simulink model "IEEE9Buses"  (R2024b)
settings: Solver=FixedStepAuto  StartTime=0  StopTime=5  FixedStep=1e-6  RelTol=1e-3
values from neighbouring files (symbols this model uses):
  SG_D_1_D = 0.01056    [SG9_parameters.m]
  SG_D_1_EnableSaturation = 0    [SG9_parameters.m]
  SG_D_1_f0 = 60    [SG9_parameters.m]
  SG_D_1_H = 7.5    [SG9_parameters.m]
  SG_D_1_K_A = 20    [SG9_parameters.m]
  SG_D_1_K_E = 1.000000e+1    (= 10)    [SG9_parameters.m]
  SG_D_1_K_F = 2.363    [SG9_parameters.m]
  SG_D_1_K_s = 5    [SG9_parameters.m]
  SG_D_1_R_a = 0.001088    [SG9_parameters.m]
  SG_D_1_S_A = 1    [SG9_parameters.m]
  SG_D_1_S_B = 0.103    [SG9_parameters.m]
  SG_D_1_S_N = 10.659857    [SG9_parameters.m]
  SG_D_1_SpeedPara = 200    [SG9_parameters.m]
  SG_D_1_T_0 = 0.720173    [SG9_parameters.m]
  SG_D_1_T_1 = 0.3    [SG9_parameters.m]
  SG_D_1_T_2 = 0.05    [SG9_parameters.m]
  SG_D_1_T_3 = 0.02    [SG9_parameters.m]
  SG_D_1_T_4 = 0.005    [SG9_parameters.m]
  SG_D_1_T_A = 0.02    [SG9_parameters.m]
  SG_D_1_T_dd = 8.000000e+0    (= 8)    [SG9_parameters.m]
  SG_D_1_T_ddd = 0.04    [SG9_parameters.m]
  SG_D_1_T_E = 0.314    [SG9_parameters.m]
  SG_D_1_T_F = 0.35    [SG9_parameters.m]
  SG_D_1_T_qd = 0.8    [SG9_parameters.m]
  SG_D_1_T_qdd = 0.02    [SG9_parameters.m]
  SG_D_1_T_speed = 0.1    [SG9_parameters.m]
  SG_D_1_T_w = 0.5    [SG9_parameters.m]
  SG_D_1_V_ref = 1.990276    [SG9_parameters.m]
  SG_D_1_w_ref = 376.991118    [SG9_parameters.m]
  SG_D_1_x_d = 1.9    [SG9_parameters.m]
  SG_D_1_x_dd = 0.302    [SG9_parameters.m]
  SG_D_1_x_ddd = 0.204    [SG9_parameters.m]
  SG_D_1_x_l = 0.05    [SG9_parameters.m]
  SG_D_1_x_q = 1.3    [SG9_parameters.m]
  SG_D_1_x_qd = 0.5    [SG9_parameters.m]
  SG_D_1_x_qdd = 0.3    [SG9_parameters.m]
  SG_D_2_D = 0.01056    [SG9_parameters.m]
  SG_D_2_EnableSaturation = 0    [SG9_parameters.m]
  SG_D_2_f0 = 60    [SG9_parameters.m]
  SG_D_2_H = 7.5    [SG9_parameters.m]
  SG_D_2_K_A = 20    [SG9_parameters.m]
  SG_D_2_K_E = 1.000000e+1    (= 10)    [SG9_parameters.m]
  SG_D_2_K_F = 2.363    [SG9_parameters.m]
  SG_D_2_K_s = 0.5    [SG9_parameters.m]
  SG_D_2_R_a = 0.001088    [SG9_parameters.m]
  SG_D_2_S_A = 1    [SG9_parameters.m]
  SG_D_2_S_B = 0.103    [SG9_parameters.m]
  SG_D_2_S_N = 10.659857    [SG9_parameters.m]
  SG_D_2_SpeedPara = 200    [SG9_parameters.m]
  SG_D_2_T_0 = 1.632913    [SG9_parameters.m]
  SG_D_2_T_1 = 0.2    [SG9_parameters.m]
  SG_D_2_T_2 = 0.05    [SG9_parameters.m]
  SG_D_2_T_3 = 0.02    [SG9_parameters.m]
  SG_D_2_T_4 = 0.005    [SG9_parameters.m]
  SG_D_2_T_A = 0.02    [SG9_parameters.m]
  SG_D_2_T_dd = 8.000000e+0    (= 8)    [SG9_parameters.m]
  SG_D_2_T_ddd = 0.04    [SG9_parameters.m]
  SG_D_2_T_E = 0.314    [SG9_parameters.m]
  SG_D_2_T_F = 0.35    [SG9_parameters.m]
  SG_D_2_T_qd = 0.8    [SG9_parameters.m]
  SG_D_2_T_qdd = 0.02    [SG9_parameters.m]
  SG_D_2_T_speed = 0.1    [SG9_parameters.m]
  SG_D_2_T_w = 0.5    [SG9_parameters.m]
  SG_D_2_V_ref = 2.662631    [SG9_parameters.m]
  SG_D_2_w_ref = 376.991118    [SG9_parameters.m]
  SG_D_2_x_d = 1.9    [SG9_parameters.m]
  SG_D_2_x_dd = 0.302    [SG9_parameters.m]
  SG_D_2_x_ddd = 0.204    [SG9_parameters.m]
  SG_D_2_x_l = 0.05    [SG9_parameters.m]
  SG_D_2_x_q = 1.3    [SG9_parameters.m]
  SG_D_2_x_qd = 0.5    [SG9_parameters.m]
  SG_D_2_x_qdd = 0.3    [SG9_parameters.m]
  SG_D_3_D = 0.01056    [SG9_parameters.m]
  SG_D_3_EnableSaturation = 0    [SG9_parameters.m]
  SG_D_3_f0 = 60    [SG9_parameters.m]
  SG_D_3_H = 7.5    [SG9_parameters.m]
  SG_D_3_K_A = 20    [SG9_parameters.m]
  SG_D_3_K_E = 1.000000e+1    (= 10)    [SG9_parameters.m]
  SG_D_3_K_F = 2.363    [SG9_parameters.m]
  SG_D_3_K_s = 0.5    [SG9_parameters.m]
  SG_D_3_R_a = 0.001088    [SG9_parameters.m]
  SG_D_3_S_A = 1    [SG9_parameters.m]
  SG_D_3_S_B = 0.103    [SG9_parameters.m]
  SG_D_3_S_N = 10.659857    [SG9_parameters.m]
  SG_D_3_SpeedPara = 200    [SG9_parameters.m]
  SG_D_3_T_0 = 0.850788    [SG9_parameters.m]
  SG_D_3_T_1 = 0.2    [SG9_parameters.m]
  SG_D_3_T_2 = 0.05    [SG9_parameters.m]
  SG_D_3_T_3 = 0.02    [SG9_parameters.m]
  SG_D_3_T_4 = 0.005    [SG9_parameters.m]
  SG_D_3_T_A = 0.02    [SG9_parameters.m]
  SG_D_3_T_dd = 8.000000e+0    (= 8)    [SG9_parameters.m]
  SG_D_3_T_ddd = 0.04    [SG9_parameters.m]
  SG_D_3_T_E = 0.314    [SG9_parameters.m]
  SG_D_3_T_F = 0.35    [SG9_parameters.m]
  SG_D_3_T_qd = 0.8    [SG9_parameters.m]
  SG_D_3_T_qdd = 0.02    [SG9_parameters.m]
  SG_D_3_T_speed = 0.1    [SG9_parameters.m]
  SG_D_3_T_w = 0.5    [SG9_parameters.m]
  SG_D_3_V_ref = 1.915682    [SG9_parameters.m]
  SG_D_3_w_ref = 376.991118    [SG9_parameters.m]
  SG_D_3_x_d = 1.9    [SG9_parameters.m]
  SG_D_3_x_dd = 0.302    [SG9_parameters.m]
  SG_D_3_x_ddd = 0.204    [SG9_parameters.m]
  SG_D_3_x_l = 0.05    [SG9_parameters.m]
  SG_D_3_x_q = 1.3    [SG9_parameters.m]
  SG_D_3_x_qd = 0.5    [SG9_parameters.m]
  SG_D_3_x_qdd = 0.3    [SG9_parameters.m]
(part 7 of 9)

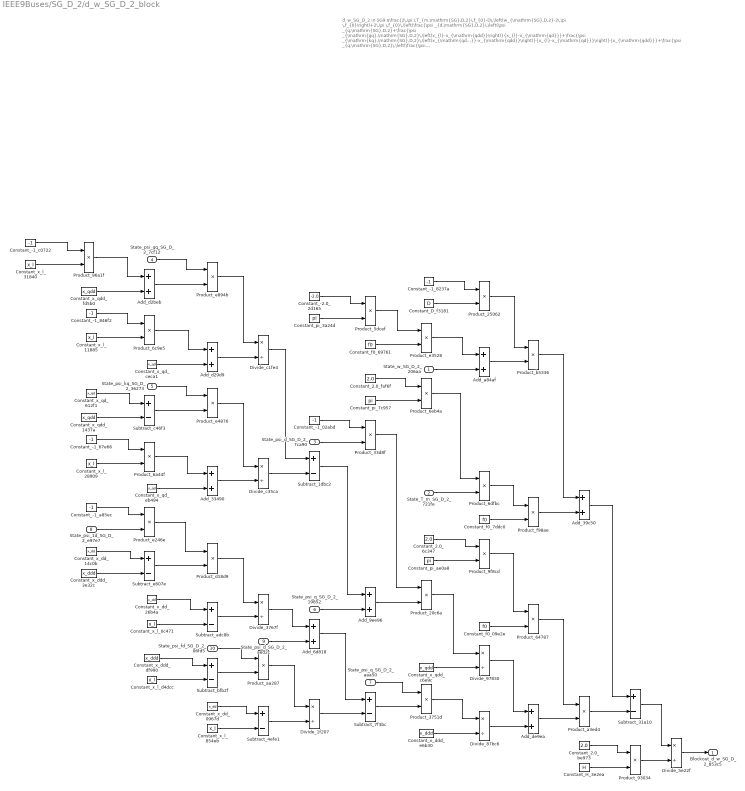
== system IEEE9Buses/SG_D_2/d_w_SG_D_2_block ==
  note: d_w_SG_D_2 in SG9
      | $\frac{2\,\pi \,T_{m,\mathrm{SG},D,2}\,f_{0}-D\,\left(w_{\mathrm{SG},D,2}-2\,\pi \,f_{0}\right)+2\,\pi \,f_{0}\,\left(\frac{\psi _{d,\mathrm{SG},D,2}\,\left(\psi _{q,\mathrm{SG},D,2}+\frac{\psi _{\mathrm{gq},\mathrm{SG},D,2}\,\left(x_{l}-x_{\mathrm{qdd}}\right)}{x_{l}-x_{\mathrm{qd}}}+\frac{\psi _{\mathrm{kq},\mathrm{SG},D,2}\,\left(x_{\mathrm{qd}}-x_{\mathrm{qdd}}\right)}{x_{l}-x_{\mathrm{qd}}}\right)}{x_{\mathrm{qdd}}}+\frac{\psi _{q,\mathrm{SG},D,2}\,\left(\frac{\psi _{\mathrm{1d},\mathrm{SG},D,2}\,\left(x_{\mathrm{dd}}-x_{\mathrm{ddd}}\right)}{x_{\mathrm{dd}}-x_{l}}-\psi _{d,\mathrm{SG},D,2}+\frac{\psi _{\mathrm{fd},\mathrm{SG},D,2}\,\left(x_{\mathrm{ddd}}-x_{l}\right)}{x_{\mathrm{dd}}-x_{l}}\right)}{x_{\mathrm{ddd}}}\right)}{2\,H}$
      | Automatically generated on 2025-09-12 21:32:25 .
  State_w_SG_D_2_206aa : Inport
  State_T_m_SG_D_2_721fe : Inport  Port=2
  State_psi_d_SG_D_2_7ca90 : Inport  Port=3
  State_psi_gq_SG_D_2_7cf12 : Inport  Port=4
  State_psi_kq_SG_D_2_36273 : Inport  Port=5
  State_psi_q_SG_D_2_19852 : Inport  Port=6
  State_psi_q_SG_D_2_aaa50 : Inport  Port=7
  State_psi_1d_SG_D_2_e97e7 : Inport  Port=8
  State_psi_d_SG_D_2_aed2c : Inport  Port=9
  State_psi_fd_SG_D_2_06fd5 : Inport  Port=10
  Add_33490 : Sum
  Add_39c50 : Sum
  Add_6d818 : Sum
  Add_9ee96 : Sum
  Add_a84af : Sum
  Add_d29d9 : Sum
  Add_d2beb : Sum
  Add_de9ea : Sum
  Constant_-1_02abd : Constant  Value=-1
  Constant_-1_67e66 : Constant  Value=-1
  Constant_-1_8237a : Constant  Value=-1
  Constant_-1_846f2 : Constant  Value=-1
  Constant_-1_a85ec : Constant  Value=-1
  Constant_-1_c0722 : Constant  Value=-1
  Constant_-2.0_2d165 : Constant  Value=-2.0
  Constant_2.0_6c347 : Constant  Value=2.0
  Constant_2.0_be973 : Constant  Value=2.0
  Constant_2.0_faf6f : Constant  Value=2.0
  Constant_D_f3181 : Constant  Value=D
  Constant_H_3e2ea : Constant  Value=H
  Constant_f0_09e2e : Constant  Value=f0
  Constant_f0_69761 : Constant  Value=f0
  Constant_f0_7ddc0 : Constant  Value=f0
  Constant_pi_3a24d : Constant  Value=pi
  Constant_pi_7c957 : Constant  Value=pi
  Constant_pi_ae0a8 : Constant  Value=pi
  Constant_x_dd_0967d : Constant  Value=x_dd
  Constant_x_dd_14c0b : Constant  Value=x_dd
  Constant_x_dd_26b4a : Constant  Value=x_dd
  Constant_x_ddd_3e32c : Constant  Value=x_ddd
  Constant_x_ddd_df990 : Constant  Value=x_ddd
  Constant_x_ddd_e6b30 : Constant  Value=x_ddd
  Constant_x_l_0c471 : Constant  Value=x_l
  Constant_x_l_11885 : Constant  Value=x_l
  Constant_x_l_28909 : Constant  Value=x_l
  Constant_x_l_31840 : Constant  Value=x_l
  Constant_x_l_854eb : Constant  Value=x_l
  Constant_x_l_d4dcc : Constant  Value=x_l
  Constant_x_qd_612f1 : Constant  Value=x_qd
  Constant_x_qd_ceca1 : Constant  Value=x_qd
  Constant_x_qd_eb494 : Constant  Value=x_qd
  Constant_x_qdd_1437a : Constant  Value=x_qdd
  Constant_x_qdd_c6e9c : Constant  Value=x_qdd
  Constant_x_qdd_fd5b0 : Constant  Value=x_qdd
  Divide_1f207 : Product  Inputs=*/
  Divide_3767f : Product  Inputs=*/
  Divide_5e22f : Product  Inputs=*/
  Divide_87bc6 : Product  Inputs=*/
  Divide_97830 : Product  Inputs=*/
  Divide_c1fe4 : Product  Inputs=*/
  Divide_c35ca : Product  Inputs=*/
  Product_20c6a : Product
  Product_25062 : Product
  Product_33d8f : Product
  Product_3751d : Product
  Product_5dcef : Product
  Product_64787 : Product
  Product_6a44f : Product
  Product_6c9e5 : Product
  Product_6dfbc : Product
  Product_6eb4a : Product
  Product_93034 : Product
  Product_96a1f : Product
  Product_9f8cd : Product
  Product_a3ed4 : Product
  Product_aa287 : Product
  Product_b5336 : Product
  Product_d18d9 : Product
  Product_e246e : Product
  Product_e3528 : Product
  Product_e4876 : Product
  Product_e894b : Product
  Product_f98ae : Product
  Subtract_1dbc2 : Sum  Inputs=+-
  Subtract_31a10 : Sum  Inputs=+-
  Subtract_4efe1 : Sum  Inputs=+-
  Subtract_7f3bc : Sum  Inputs=+-
  Subtract_adc8b : Sum  Inputs=+-
  Subtract_bfb2f : Sum  Inputs=+-
  Subtract_c46f3 : Sum  Inputs=+-
  Subtract_e607e : Sum  Inputs=+-
  Blockout_d_w_SG_D_2_853c5 : Outport
  wires:
  Constant_x_qd_612f1/1 -> Subtract_c46f3/1
  Constant_-1_67e66/1 -> Product_6a44f/1
  Constant_-1_c0722/1 -> Product_96a1f/1
  Constant_x_qdd_1437a/1 -> Subtract_c46f3/2
  Subtract_4efe1/1 -> Divide_1f207/2
  Constant_x_l_28909/1 -> Product_6a44f/2
  Constant_x_l_31840/1 -> Product_96a1f/2
  Product_6a44f/1 -> Add_33490/1
  Product_96a1f/1 -> Add_d2beb/1
  Constant_x_l_0c471/1 -> Subtract_adc8b/2
  Constant_x_l_11885/1 -> Product_6c9e5/2
  Constant_x_ddd_e6b30/1 -> Divide_87bc6/2
  Subtract_bfb2f/1 -> Product_aa287/2
  Constant_x_qd_eb494/1 -> Add_33490/2
  Constant_x_qdd_fd5b0/1 -> Add_d2beb/2
  Constant_-1_846f2/1 -> Product_6c9e5/1
  State_psi_d_SG_D_2_7ca90/1 -> Product_33d8f/2
  Constant_-1_a85ec/1 -> Product_e246e/1
  State_w_SG_D_2_206aa/1 -> Add_a84af/2
  Product_6c9e5/1 -> Add_d29d9/1
  State_psi_1d_SG_D_2_e97e7/1 -> Product_e246e/2
  Constant_x_dd_14c0b/1 -> Subtract_e607e/1
  Divide_c1fe4/1 -> Subtract_1dbc2/1
  Subtract_c46f3/1 -> Product_e4876/2
  Constant_x_ddd_3e32c/1 -> Subtract_e607e/2
  State_psi_gq_SG_D_2_7cf12/1 -> Product_e894b/1
  Add_33490/1 -> Divide_c35ca/2
  State_psi_d_SG_D_2_aed2c/1 -> Add_6d818/2
  Add_d2beb/1 -> Product_e894b/2
  Constant_x_qd_ceca1/1 -> Add_d29d9/2
  State_psi_kq_SG_D_2_36273/1 -> Product_e4876/1
  Product_e246e/1 -> Product_d18d9/1
  Subtract_e607e/1 -> Product_d18d9/2
  Constant_pi_7c957/1 -> Product_6eb4a/2
  Constant_x_dd_26b4a/1 -> Subtract_adc8b/1
  Constant_x_ddd_df990/1 -> Subtract_bfb2f/1
  Constant_x_l_d4dcc/1 -> Subtract_bfb2f/2
  Product_e894b/1 -> Divide_c1fe4/1
  Add_d29d9/1 -> Divide_c1fe4/2
  Add_9ee96/1 -> Product_20c6a/2
  Product_e4876/1 -> Divide_c35ca/1
  Constant_pi_3a24d/1 -> Product_5dcef/2
  Product_d18d9/1 -> Divide_3767f/1
  Subtract_adc8b/1 -> Divide_3767f/2
  State_psi_fd_SG_D_2_06fd5/1 -> Product_aa287/1
  Divide_3767f/1 -> Add_6d818/1
  Constant_x_dd_0967d/1 -> Subtract_4efe1/1
  Constant_x_l_854eb/1 -> Subtract_4efe1/2
  Divide_c35ca/1 -> Subtract_1dbc2/2
  Product_aa287/1 -> Divide_1f207/1
  Constant_-1_02abd/1 -> Product_33d8f/1
  Constant_-2.0_2d165/1 -> Product_5dcef/1
  Subtract_1dbc2/1 -> Add_9ee96/1
  Subtract_7f3bc/1 -> Product_3751d/2
  State_psi_q_SG_D_2_19852/1 -> Add_9ee96/2
  Constant_D_f3181/1 -> Product_25062/2
  Add_6d818/1 -> Subtract_7f3bc/1
  Divide_1f207/1 -> Subtract_7f3bc/2
  Product_5dcef/1 -> Product_e3528/1
  Constant_f0_69761/1 -> Product_e3528/2
  Constant_2.0_faf6f/1 -> Product_6eb4a/1
  Product_33d8f/1 -> Product_20c6a/1
  State_psi_q_SG_D_2_aaa50/1 -> Product_3751d/1
  Constant_-1_8237a/1 -> Product_25062/1
  Product_e3528/1 -> Add_a84af/1
  Product_6eb4a/1 -> Product_6dfbc/1
  State_T_m_SG_D_2_721fe/1 -> Product_6dfbc/2
  Constant_2.0_6c347/1 -> Product_9f8cd/1
  Constant_pi_ae0a8/1 -> Product_9f8cd/2
  Product_20c6a/1 -> Divide_97830/1
  Constant_x_qdd_c6e9c/1 -> Divide_97830/2
  Product_3751d/1 -> Divide_87bc6/1
  Product_25062/1 -> Product_b5336/1
  Add_a84af/1 -> Product_b5336/2
  Product_6dfbc/1 -> Product_f98ae/1
  Constant_f0_7ddc0/1 -> Product_f98ae/2
  Product_9f8cd/1 -> Product_64787/1
  Constant_f0_09e2e/1 -> Product_64787/2
  Divide_97830/1 -> Add_de9ea/1
  Divide_87bc6/1 -> Add_de9ea/2
  Product_b5336/1 -> Add_39c50/1
  Product_f98ae/1 -> Add_39c50/2
  Product_64787/1 -> Product_a3ed4/1
  Add_de9ea/1 -> Product_a3ed4/2
  Add_39c50/1 -> Subtract_31a10/1
  Product_a3ed4/1 -> Subtract_31a10/2
  Constant_2.0_be973/1 -> Product_93034/1
  Constant_H_3e2ea/1 -> Product_93034/2
  Subtract_31a10/1 -> Divide_5e22f/1
  Product_93034/1 -> Divide_5e22f/2
  Divide_5e22f/1 -> Blockout_d_w_SG_D_2_853c5/1

== system IEEE9Buses/SG_D_2/i_d_SG_D_2_block ==
  note: i_d_SG_D_2 in SG9
      | $\frac{\sin\left(\theta _{\mathrm{SG},D,2}\right)\,\left(\frac{\psi _{\mathrm{1d},\mathrm{SG},D,2}\,\left(x_{\mathrm{dd}}-x_{\mathrm{ddd}}\right)}{x_{\mathrm{dd}}-x_{l}}-\psi _{d,\mathrm{SG},D,2}+\frac{\psi _{\mathrm{fd},\mathrm{SG},D,2}\,\left(x_{\mathrm{ddd}}-x_{l}\right)}{x_{\mathrm{dd}}-x_{l}}\right)}{x_{\mathrm{ddd}}}-\frac{\cos\left(\theta _{\mathrm{SG},D,2}\right)\,\left(\psi _{q,\mathrm{SG},D,2}+\frac{\psi _{\mathrm{gq},\mathrm{SG},D,2}\,\left(x_{l}-x_{\mathrm{qdd}}\right)}{x_{l}-x_{\mathrm{qd}}}+\frac{\psi _{\mathrm{kq},\mathrm{SG},D,2}\,\left(x_{\mathrm{qd}}-x_{\mathrm{qdd}}\right)}{x_{l}-x_{\mathrm{qd}}}\right)}{x_{\mathrm{qdd}}}$
      | Automatically generated on 2025-09-12 21:32:46 .
  State_psi_gq_SG_D_2_90053 : Inport
  State_psi_kq_SG_D_2_eb372 : Inport  Port=2
  State_psi_q_SG_D_2_21c3a : Inport  Port=3
  State_theta_SG_D_2_ad8b9 : Inport  Port=4
  State_psi_1d_SG_D_2_6831d : Inport  Port=5
  State_psi_d_SG_D_2_b6ace : Inport  Port=6
  State_psi_fd_SG_D_2_d29ae : Inport  Port=7
  State_theta_SG_D_2_d994c : Inport  Port=8
  Add_2b227 : Sum
  Add_62690 : Sum
  Add_a08b0 : Sum
  Add_f95a1 : Sum
  Add_fd884 : Sum
  Constant_-1_06c4e : Constant  Value=-1
  Constant_-1_18421 : Constant  Value=-1
  Constant_-1_9588e : Constant  Value=-1
  Constant_-1_961c2 : Constant  Value=-1
  Constant_-1_b9742 : Constant  Value=-1
  Constant_x_dd_735c8 : Constant  Value=x_dd
  Constant_x_dd_a57c2 : Constant  Value=x_dd
  Constant_x_dd_fe2f1 : Constant  Value=x_dd
  Constant_x_ddd_39529 : Constant  Value=x_ddd
  Constant_x_ddd_51cac : Constant  Value=x_ddd
  Constant_x_ddd_586e4 : Constant  Value=x_ddd
  Constant_x_l_46ee8 : Constant  Value=x_l
  Constant_x_l_505f4 : Constant  Value=x_l
  Constant_x_l_5ae3b : Constant  Value=x_l
  Constant_x_l_7b25a : Constant  Value=x_l
  Constant_x_l_9cc34 : Constant  Value=x_l
  Constant_x_l_ca148 : Constant  Value=x_l
  Constant_x_qd_1e2ec : Constant  Value=x_qd
  Constant_x_qd_7308e : Constant  Value=x_qd
  Constant_x_qd_f38dc : Constant  Value=x_qd
  Constant_x_qdd_2b118 : Constant  Value=x_qdd
  Constant_x_qdd_3372b : Constant  Value=x_qdd
  Constant_x_qdd_833b8 : Constant  Value=x_qdd
  Divide_5c815 : Product  Inputs=*/
  Divide_798bb : Product  Inputs=*/
  Divide_9c951 : Product  Inputs=*/
  Divide_bc0c7 : Product  Inputs=*/
  Divide_e14bd : Product  Inputs=*/
  Divide_e1946 : Product  Inputs=*/
  MathFunc_cos_20c10 : Trigonometry  Operator=cos
  MathFunc_sin_69d7d : Trigonometry
  Product_03c49 : Product
  Product_468f1 : Product
  Product_58bb8 : Product
  Product_5dc22 : Product
  Product_63187 : Product
  Product_7083f : Product
  Product_81fa6 : Product
  Product_89e84 : Product
  Product_cca34 : Product
  Product_e0f2d : Product
  Product_f1839 : Product
  Subtract_05f06 : Sum  Inputs=+-
  Subtract_10155 : Sum  Inputs=+-
  Subtract_228a0 : Sum  Inputs=+-
  Subtract_2c410 : Sum  Inputs=+-
  Subtract_57970 : Sum  Inputs=+-
  Subtract_b0f61 : Sum  Inputs=+-
  Subtract_c9259 : Sum  Inputs=+-
  Subtract_f9ac3 : Sum  Inputs=+-
  Blockout_i_d_SG_D_2_44cd5 : Outport
  wires:
  Constant_x_ddd_39529/1 -> Subtract_57970/1
  Constant_x_qd_7308e/1 -> Subtract_228a0/1
  Constant_-1_18421/1 -> Product_7083f/1
  Constant_-1_06c4e/1 -> Product_89e84/1
  Subtract_c9259/1 -> Blockout_i_d_SG_D_2_44cd5/1
  Constant_x_qdd_3372b/1 -> Subtract_228a0/2
  Constant_x_l_5ae3b/1 -> Product_7083f/2
  Constant_x_l_ca148/1 -> Product_89e84/2
  Product_7083f/1 -> Add_f95a1/1
  Product_89e84/1 -> Add_62690/1
  Constant_x_l_46ee8/1 -> Product_63187/2
  Constant_x_qd_f38dc/1 -> Add_f95a1/2
  Constant_x_qdd_833b8/1 -> Add_62690/2
  Constant_x_qdd_2b118/1 -> Divide_e1946/2
  MathFunc_cos_20c10/1 -> Product_468f1/2
  Constant_-1_961c2/1 -> Product_63187/1
  State_psi_gq_SG_D_2_90053/1 -> Product_f1839/1
  Subtract_57970/1 -> Product_cca34/2
  Product_58bb8/1 -> Product_e0f2d/1
  Add_f95a1/1 -> Divide_5c815/2
  Add_62690/1 -> Product_f1839/2
  Product_cca34/1 -> Divide_e14bd/1
  Product_63187/1 -> Add_fd884/1
  Constant_x_qd_1e2ec/1 -> Add_fd884/2
  State_theta_SG_D_2_d994c/1 -> MathFunc_sin_69d7d/1
  State_psi_kq_SG_D_2_eb372/1 -> Product_03c49/1
  Add_a08b0/1 -> Subtract_f9ac3/1
  Subtract_228a0/1 -> Product_03c49/2
  Product_f1839/1 -> Divide_798bb/1
  Constant_-1_b9742/1 -> Product_58bb8/1
  State_psi_1d_SG_D_2_6831d/1 -> Product_58bb8/2
  State_psi_fd_SG_D_2_d29ae/1 -> Product_cca34/1
  Constant_x_dd_a57c2/1 -> Subtract_2c410/1
  Product_e0f2d/1 -> Divide_bc0c7/1
  Constant_x_ddd_51cac/1 -> Subtract_2c410/2
  Divide_e14bd/1 -> Subtract_f9ac3/2
  Add_fd884/1 -> Divide_798bb/2
  Product_5dc22/1 -> Divide_9c951/1
  Product_03c49/1 -> Divide_5c815/1
  Constant_-1_9588e/1 -> Product_81fa6/1
  Subtract_b0f61/1 -> Divide_e14bd/2
  Subtract_2c410/1 -> Product_e0f2d/2
  Constant_x_dd_735c8/1 -> Subtract_10155/1
  Subtract_f9ac3/1 -> Product_5dc22/1
  Constant_x_l_9cc34/1 -> Subtract_10155/2
  Constant_x_l_505f4/1 -> Subtract_57970/2
  Divide_798bb/1 -> Subtract_05f06/1
  Divide_9c951/1 -> Subtract_c9259/2
  Divide_5c815/1 -> Subtract_05f06/2
  Subtract_10155/1 -> Divide_bc0c7/2
  Constant_x_dd_fe2f1/1 -> Subtract_b0f61/1
  Divide_e1946/1 -> Subtract_c9259/1
  Constant_x_l_7b25a/1 -> Subtract_b0f61/2
  Subtract_05f06/1 -> Add_2b227/1
  State_psi_q_SG_D_2_21c3a/1 -> Add_2b227/2
  Constant_x_ddd_586e4/1 -> Divide_9c951/2
  MathFunc_sin_69d7d/1 -> Product_5dc22/2
  Divide_bc0c7/1 -> Add_a08b0/1
  State_psi_d_SG_D_2_b6ace/1 -> Add_a08b0/2
  Add_2b227/1 -> Product_81fa6/2
  State_theta_SG_D_2_ad8b9/1 -> MathFunc_cos_20c10/1
  Product_81fa6/1 -> Product_468f1/1
  Product_468f1/1 -> Divide_e1946/1

== system IEEE9Buses/SG_D_2/i_q_SG_D_2_block ==
  note: i_q_SG_D_2 in SG9
      | $-\frac{\sin\left(\theta _{\mathrm{SG},D,2}\right)\,\left(\psi _{q,\mathrm{SG},D,2}+\frac{\psi _{\mathrm{gq},\mathrm{SG},D,2}\,\left(x_{l}-x_{\mathrm{qdd}}\right)}{x_{l}-x_{\mathrm{qd}}}+\frac{\psi _{\mathrm{kq},\mathrm{SG},D,2}\,\left(x_{\mathrm{qd}}-x_{\mathrm{qdd}}\right)}{x_{l}-x_{\mathrm{qd}}}\right)}{x_{\mathrm{qdd}}}-\frac{\cos\left(\theta _{\mathrm{SG},D,2}\right)\,\left(\frac{\psi _{\mathrm{1d},\mathrm{SG},D,2}\,\left(x_{\mathrm{dd}}-x_{\mathrm{ddd}}\right)}{x_{\mathrm{dd}}-x_{l}}-\psi _{d,\mathrm{SG},D,2}+\frac{\psi _{\mathrm{fd},\mathrm{SG},D,2}\,\left(x_{\mathrm{ddd}}-x_{l}\right)}{x_{\mathrm{dd}}-x_{l}}\right)}{x_{\mathrm{ddd}}}$
      | Automatically generated on 2025-09-12 21:32:49 .
  State_psi_gq_SG_D_2_3847f : Inport
  State_psi_kq_SG_D_2_83339 : Inport  Port=2
  State_psi_q_SG_D_2_adea4 : Inport  Port=3
  State_theta_SG_D_2_b1bab : Inport  Port=4
  State_psi_1d_SG_D_2_91d23 : Inport  Port=5
  State_psi_d_SG_D_2_186b2 : Inport  Port=6
  State_psi_fd_SG_D_2_f955d : Inport  Port=7
  State_theta_SG_D_2_88755 : Inport  Port=8
  Add_10559 : Sum
  Add_41a96 : Sum
  Add_72399 : Sum
  Add_88e3a : Sum
  Add_bf917 : Sum
  Add_f05d7 : Sum
  Constant_-1_37a87 : Constant  Value=-1
  Constant_-1_4223b : Constant  Value=-1
  Constant_-1_5e843 : Constant  Value=-1
  Constant_-1_e87cb : Constant  Value=-1
  Constant_-1_e91bf : Constant  Value=-1
  Constant_x_dd_2cca8 : Constant  Value=x_dd
  Constant_x_dd_6db02 : Constant  Value=x_dd
  Constant_x_dd_7201c : Constant  Value=x_dd
  Constant_x_ddd_02ef5 : Constant  Value=x_ddd
  Constant_x_ddd_35ad7 : Constant  Value=x_ddd
  Constant_x_ddd_b63ec : Constant  Value=x_ddd
  Constant_x_l_537d7 : Constant  Value=x_l
  Constant_x_l_6cc43 : Constant  Value=x_l
  Constant_x_l_83442 : Constant  Value=x_l
  Constant_x_l_9a67a : Constant  Value=x_l
  Constant_x_l_9c9f6 : Constant  Value=x_l
  Constant_x_l_c45e2 : Constant  Value=x_l
  Constant_x_qd_59276 : Constant  Value=x_qd
  Constant_x_qd_b17a7 : Constant  Value=x_qd
  Constant_x_qd_f3cf5 : Constant  Value=x_qd
  Constant_x_qdd_3f35f : Constant  Value=x_qdd
  Constant_x_qdd_c06d0 : Constant  Value=x_qdd
  Constant_x_qdd_ddfed : Constant  Value=x_qdd
  Divide_01780 : Product  Inputs=*/
  Divide_28376 : Product  Inputs=*/
  Divide_330b8 : Product  Inputs=*/
  Divide_352e0 : Product  Inputs=*/
  Divide_42aad : Product  Inputs=*/
  Divide_7f640 : Product  Inputs=*/
  MathFunc_cos_f641c : Trigonometry  Operator=cos
  MathFunc_sin_d2e3f : Trigonometry
  Product_0c9e1 : Product
  Product_19aca : Product
  Product_2429a : Product
  Product_25fd3 : Product
  Product_351b7 : Product
  Product_3777c : Product
  Product_529ed : Product
  Product_84d7b : Product
  Product_889bc : Product
  Product_da850 : Product
  Product_fe36e : Product
  Subtract_486ae : Sum  Inputs=+-
  Subtract_69592 : Sum  Inputs=+-
  Subtract_8fc73 : Sum  Inputs=+-
  Subtract_b660b : Sum  Inputs=+-
  Subtract_d2259 : Sum  Inputs=+-
  Subtract_daa1e : Sum  Inputs=+-
  Subtract_fe410 : Sum  Inputs=+-
  Blockout_i_q_SG_D_2_7be03 : Outport
  wires:
  MathFunc_sin_d2e3f/1 -> Product_889bc/2
  Product_fe36e/1 -> Product_889bc/1
  Constant_-1_37a87/1 -> Product_da850/1
  Constant_-1_e91bf/1 -> Product_351b7/1
  Constant_x_l_c45e2/1 -> Product_da850/2
  Product_da850/1 -> Add_41a96/1
  Subtract_d2259/1 -> Product_529ed/2
  Constant_x_qdd_3f35f/1 -> Subtract_daa1e/2
  Constant_x_qdd_c06d0/1 -> Add_41a96/2
  Add_88e3a/1 -> Product_fe36e/2
  Constant_x_l_9c9f6/1 -> Product_351b7/2
  Constant_x_qd_59276/1 -> Subtract_daa1e/1
  Constant_-1_4223b/1 -> Product_0c9e1/1
  Constant_x_l_537d7/1 -> Product_0c9e1/2
  State_psi_1d_SG_D_2_91d23/1 -> Product_84d7b/2
  State_psi_gq_SG_D_2_3847f/1 -> Product_2429a/1
  Add_41a96/1 -> Product_2429a/2
  Product_351b7/1 -> Add_f05d7/1
  Divide_42aad/1 -> Add_10559/1
  Constant_x_qd_f3cf5/1 -> Add_f05d7/2
  State_psi_kq_SG_D_2_83339/1 -> Product_25fd3/1
  Add_72399/1 -> Subtract_8fc73/1
  Constant_x_ddd_02ef5/1 -> Subtract_d2259/2
  Subtract_daa1e/1 -> Product_25fd3/2
  Product_0c9e1/1 -> Add_bf917/1
  Constant_x_qd_b17a7/1 -> Add_bf917/2
  Constant_-1_5e843/1 -> Product_84d7b/1
  Constant_x_l_83442/1 -> Subtract_69592/2
  Constant_x_dd_6db02/1 -> Subtract_d2259/1
  Product_2429a/1 -> Divide_28376/1
  Divide_330b8/1 -> Subtract_8fc73/2
  Add_f05d7/1 -> Divide_28376/2
  Product_3777c/1 -> Divide_352e0/1
  Product_25fd3/1 -> Divide_7f640/1
  Constant_-1_e87cb/1 -> Product_fe36e/1
  Product_84d7b/1 -> Product_529ed/1
  Add_bf917/1 -> Divide_7f640/2
  Constant_x_dd_2cca8/1 -> Subtract_486ae/1
  Subtract_8fc73/1 -> Product_3777c/1
  Subtract_fe410/1 -> Product_19aca/2
  Constant_x_l_6cc43/1 -> Subtract_486ae/2
  Constant_x_ddd_b63ec/1 -> Subtract_fe410/1
  Constant_x_l_9a67a/1 -> Subtract_fe410/2
  Divide_28376/1 -> Subtract_b660b/1
  Divide_352e0/1 -> Add_10559/2
  Product_19aca/1 -> Divide_330b8/1
  Divide_7f640/1 -> Subtract_b660b/2
  Subtract_69592/1 -> Divide_330b8/2
  Product_529ed/1 -> Divide_01780/1
  Subtract_486ae/1 -> Divide_01780/2
  Constant_x_qdd_ddfed/1 -> Divide_42aad/2
  State_psi_fd_SG_D_2_f955d/1 -> Product_19aca/1
  Constant_x_dd_7201c/1 -> Subtract_69592/1
  Subtract_b660b/1 -> Add_88e3a/1
  State_psi_q_SG_D_2_adea4/1 -> Add_88e3a/2
  Constant_x_ddd_35ad7/1 -> Divide_352e0/2
  Divide_01780/1 -> Add_72399/1
  State_psi_d_SG_D_2_186b2/1 -> Add_72399/2
  State_theta_SG_D_2_b1bab/1 -> MathFunc_sin_d2e3f/1
  State_theta_SG_D_2_88755/1 -> MathFunc_cos_f641c/1
  MathFunc_cos_f641c/1 -> Product_3777c/2
  Product_889bc/1 -> Divide_42aad/1
  Add_10559/1 -> Blockout_i_q_SG_D_2_7be03/1

== system IEEE9Buses/SG_D_2/theta_SG_D_2_out_block ==
  note: theta_SG_D_2_out in SG9
      | $\theta _{\mathrm{SG},D,2}$
      | Automatically generated on 2025-09-12 21:32:54 .
  State_theta_SG_D_2_4fa63 : Inport
  Blockout_theta_SG_D_2_out_702a9 : Outport
  wires:
  State_theta_SG_D_2_4fa63/1 -> Blockout_theta_SG_D_2_out_702a9/1

== system IEEE9Buses/SG_D_2/w_SG_D_2_out_block ==
  note: w_SG_D_2_out in SG9
      | $w_{\mathrm{SG},D,2}$
      | Automatically generated on 2025-09-12 21:32:54 .
  State_w_SG_D_2_7ad77 : Inport
  Blockout_w_SG_D_2_out_8dce1 : Outport
  wires:
  State_w_SG_D_2_7ad77/1 -> Blockout_w_SG_D_2_out_8dce1/1

== system IEEE9Buses/SG_D_3/T_e_SG_D_3_block ==
  note: T_e_SG_D_3 in SG9
      | $-\frac{\psi _{d,\mathrm{SG},D,3}\,\left(\psi _{q,\mathrm{SG},D,3}+\frac{\psi _{\mathrm{gq},\mathrm{SG},D,3}\,\left(x_{l}-x_{\mathrm{qdd}}\right)}{x_{l}-x_{\mathrm{qd}}}+\frac{\psi _{\mathrm{kq},\mathrm{SG},D,3}\,\left(x_{\mathrm{qd}}-x_{\mathrm{qdd}}\right)}{x_{l}-x_{\mathrm{qd}}}\right)}{x_{\mathrm{qdd}}}-\frac{\psi _{q,\mathrm{SG},D,3}\,\left(\frac{\psi _{\mathrm{1d},\mathrm{SG},D,3}\,\left(x_{\mathrm{dd}}-x_{\mathrm{ddd}}\right)}{x_{\mathrm{dd}}-x_{l}}-\psi _{d,\mathrm{SG},D,3}+\frac{\psi _{\mathrm{fd},\mathrm{SG},D,3}\,\left(x_{\mathrm{ddd}}-x_{l}\right)}{x_{\mathrm{dd}}-x_{l}}\right)}{x_{\mathrm{ddd}}}$
      | Automatically generated on 2025-09-12 21:34:00 .
  State_psi_d_SG_D_3_17815 : Inport
  State_psi_gq_SG_D_3_9a032 : Inport  Port=2
  State_psi_kq_SG_D_3_18e1d : Inport  Port=3
  State_psi_q_SG_D_3_3fc53 : Inport  Port=4
  State_psi_q_SG_D_3_9d696 : Inport  Port=5
  State_psi_1d_SG_D_3_e0c74 : Inport  Port=6
  State_psi_d_SG_D_3_9e4e7 : Inport  Port=7
  State_psi_fd_SG_D_3_cc739 : Inport  Port=8
  Add_0e30c : Sum
  Add_10f0c : Sum
  Add_86e12 : Sum
  Add_87df8 : Sum
  Add_b72cb : Sum
  Add_f48ca : Sum
  Constant_-1_1b9c5 : Constant  Value=-1
  Constant_-1_221eb : Constant  Value=-1
  Constant_-1_85dbb : Constant  Value=-1
  Constant_-1_bd3ea : Constant  Value=-1
  Constant_-1_d71e6 : Constant  Value=-1
  Constant_x_dd_3c33d : Constant  Value=x_dd
  Constant_x_dd_a61e5 : Constant  Value=x_dd
  Constant_x_dd_d9738 : Constant  Value=x_dd
  Constant_x_ddd_65fa8 : Constant  Value=x_ddd
  Constant_x_ddd_7cd06 : Constant  Value=x_ddd
  Constant_x_ddd_a3935 : Constant  Value=x_ddd
  Constant_x_l_1ac7a : Constant  Value=x_l
  Constant_x_l_280c5 : Constant  Value=x_l
  Constant_x_l_3e38e : Constant  Value=x_l
  Constant_x_l_8e34f : Constant  Value=x_l
  Constant_x_l_cf327 : Constant  Value=x_l
  Constant_x_l_dac06 : Constant  Value=x_l
  Constant_x_qd_b1f4e : Constant  Value=x_qd
  Constant_x_qd_caa55 : Constant  Value=x_qd
  Constant_x_qd_d5515 : Constant  Value=x_qd
  Constant_x_qdd_45dd8 : Constant  Value=x_qdd
  Constant_x_qdd_d54be : Constant  Value=x_qdd
  Constant_x_qdd_e5fa9 : Constant  Value=x_qdd
  Divide_57d3c : Product  Inputs=*/
  Divide_7daa9 : Product  Inputs=*/
  Divide_901bf : Product  Inputs=*/
  Divide_97a01 : Product  Inputs=*/
  Divide_97b52 : Product  Inputs=*/
  Divide_a8233 : Product  Inputs=*/
  Product_17860 : Product
  Product_2bd1e : Product
  Product_4f0bb : Product
  Product_63321 : Product
  Product_728b3 : Product
  Product_77792 : Product
  Product_a3c9e : Product
  Product_a9e3d : Product
  Product_cb385 : Product
  Product_fbc8a : Product
  Product_fd87a : Product
  Subtract_23dbe : Sum  Inputs=+-
  Subtract_271b0 : Sum  Inputs=+-
  Subtract_3d733 : Sum  Inputs=+-
  Subtract_8448f : Sum  Inputs=+-
  Subtract_a8c5a : Sum  Inputs=+-
  Subtract_ad38a : Sum  Inputs=+-
  Subtract_e1daa : Sum  Inputs=+-
  Blockout_T_e_SG_D_3_2b576 : Outport
  wires:
  State_psi_q_SG_D_3_3fc53/1 -> Add_10f0c/2
  Constant_-1_bd3ea/1 -> Product_cb385/1
  Subtract_23dbe/1 -> Product_17860/2
  State_psi_1d_SG_D_3_e0c74/1 -> Product_a3c9e/2
  Constant_-1_1b9c5/1 -> Product_4f0bb/1
  Constant_x_l_1ac7a/1 -> Product_4f0bb/2
  Add_f48ca/1 -> Subtract_23dbe/1
  State_psi_d_SG_D_3_9e4e7/1 -> Add_f48ca/2
  Product_4f0bb/1 -> Add_86e12/1
  Constant_x_qdd_e5fa9/1 -> Subtract_271b0/2
  Add_10f0c/1 -> Product_a9e3d/2
  Constant_x_qdd_45dd8/1 -> Add_86e12/2
  State_psi_q_SG_D_3_9d696/1 -> Product_17860/1
  Constant_x_l_8e34f/1 -> Product_cb385/2
  Subtract_ad38a/1 -> Divide_57d3c/2
  Constant_x_l_3e38e/1 -> Subtract_e1daa/2
  Constant_x_qd_b1f4e/1 -> Subtract_271b0/1
  Constant_-1_221eb/1 -> Product_728b3/1
  Subtract_8448f/1 -> Divide_a8233/2
  Constant_x_l_dac06/1 -> Product_728b3/2
  Product_fbc8a/1 -> Divide_a8233/1
  Constant_-1_d71e6/1 -> Product_a3c9e/1
  Product_a3c9e/1 -> Product_fbc8a/1
  Constant_x_dd_3c33d/1 -> Subtract_a8c5a/1
  Constant_x_ddd_7cd06/1 -> Subtract_a8c5a/2
  Add_0e30c/1 -> Blockout_T_e_SG_D_3_2b576/1
  State_psi_gq_SG_D_3_9a032/1 -> Product_63321/1
  Product_17860/1 -> Divide_901bf/1
  Add_86e12/1 -> Product_63321/2
  State_psi_fd_SG_D_3_cc739/1 -> Product_77792/1
  Product_cb385/1 -> Add_b72cb/1
  Constant_x_qd_caa55/1 -> Add_b72cb/2
  Constant_x_dd_a61e5/1 -> Subtract_8448f/1
  State_psi_kq_SG_D_3_18e1d/1 -> Product_fd87a/1
  Constant_x_dd_d9738/1 -> Subtract_ad38a/1
  Subtract_271b0/1 -> Product_fd87a/2
  Product_a9e3d/1 -> Divide_97b52/1
  Product_728b3/1 -> Add_87df8/1
  Add_b72cb/1 -> Divide_7daa9/2
  Constant_x_qd_d5515/1 -> Add_87df8/2
  Subtract_a8c5a/1 -> Product_fbc8a/2
  Constant_x_l_cf327/1 -> Subtract_8448f/2
  Constant_x_ddd_a3935/1 -> Subtract_e1daa/1
  Product_63321/1 -> Divide_7daa9/1
  Product_fd87a/1 -> Divide_97a01/1
  Add_87df8/1 -> Divide_97a01/2
  Constant_x_ddd_65fa8/1 -> Divide_901bf/2
  Subtract_e1daa/1 -> Product_77792/2
  Divide_7daa9/1 -> Subtract_3d733/1
  Constant_x_l_280c5/1 -> Subtract_ad38a/2
  Divide_97a01/1 -> Subtract_3d733/2
  Divide_a8233/1 -> Add_f48ca/1
  Product_77792/1 -> Divide_57d3c/1
  Constant_-1_85dbb/1 -> Product_2bd1e/1
  State_psi_d_SG_D_3_17815/1 -> Product_2bd1e/2
  Subtract_3d733/1 -> Add_10f0c/1
  Divide_57d3c/1 -> Subtract_23dbe/2
  Product_2bd1e/1 -> Product_a9e3d/1
  Constant_x_qdd_d54be/1 -> Divide_97b52/2
  Divide_97b52/1 -> Add_0e30c/1
  Divide_901bf/1 -> Add_0e30c/2

== system IEEE9Buses/SG_D_3/d_E_fd_SG_D_3_block ==
  note: d_E_fd_SG_D_3 in SG9
      | $\frac{V_{f,\mathrm{SG},D,3}-E_{\mathrm{fd},\mathrm{SG},D,3}\,K_{E}}{T_{E}}$
      | Automatically generated on 2025-09-12 21:33:44 .
  State_E_fd_SG_D_3_1d006 : Inport
  State_V_f_SG_D_3_25ca2 : Inport  Port=2
  Add_d6ece : Sum
  Constant_-1_e5d62 : Constant  Value=-1
  Constant_K_E_db232 : Constant  Value=K_E
  Constant_T_E_f9617 : Constant  Value=T_E
  Divide_8676b : Product  Inputs=*/
  Product_40125 : Product
  Product_ab3a1 : Product
  Blockout_d_E_fd_SG_D_3_8d01f : Outport
  wires:
  State_V_f_SG_D_3_25ca2/1 -> Add_d6ece/2
  Constant_-1_e5d62/1 -> Product_ab3a1/1
  State_E_fd_SG_D_3_1d006/1 -> Product_ab3a1/2
  Constant_T_E_f9617/1 -> Divide_8676b/2
  Product_ab3a1/1 -> Product_40125/1
  Product_40125/1 -> Add_d6ece/1
  Constant_K_E_db232/1 -> Product_40125/2
  Divide_8676b/1 -> Blockout_d_E_fd_SG_D_3_8d01f/1
  Add_d6ece/1 -> Divide_8676b/1

== system IEEE9Buses/SG_D_3/d_Px_1_SG_D_3_block ==
  note: d_Px_1_SG_D_3 in SG9
      | $\frac{w_{\mathrm{SG},D,3}-2\,\pi \,f_{0}}{T_{w}}-\frac{\mathrm{Px}_{1,\mathrm{SG},D,3}}{T_{w}}$
      | Automatically generated on 2025-09-12 21:33:45 .
  State_Px_1_SG_D_3_a2521 : Inport
  State_w_SG_D_3_03ebd : Inport  Port=2
  Add_75672 : Sum
  Add_91898 : Sum
  Constant_-1_d7d52 : Constant  Value=-1
  Constant_-2.0_38484 : Constant  Value=-2.0
  Constant_T_w_12eeb : Constant  Value=T_w
  Constant_T_w_8327e : Constant  Value=T_w
  Constant_f0_08397 : Constant  Value=f0
  Constant_pi_f0e36 : Constant  Value=pi
  Divide_414c5 : Product  Inputs=*/
  Divide_657cb : Product  Inputs=*/
  Product_951b3 : Product
  Product_ab4b7 : Product
  Product_d73c2 : Product
  Blockout_d_Px_1_SG_D_3_0a11a : Outport
  wires:
  Constant_f0_08397/1 -> Product_d73c2/2
  Constant_-1_d7d52/1 -> Product_951b3/1
  Constant_-2.0_38484/1 -> Product_ab4b7/1
  Constant_pi_f0e36/1 -> Product_ab4b7/2
  Product_ab4b7/1 -> Product_d73c2/1
  State_w_SG_D_3_03ebd/1 -> Add_75672/2
  Divide_657cb/1 -> Add_91898/1
  State_Px_1_SG_D_3_a2521/1 -> Product_951b3/2
  Product_d73c2/1 -> Add_75672/1
  Product_951b3/1 -> Divide_657cb/1
  Constant_T_w_8327e/1 -> Divide_657cb/2
  Add_75672/1 -> Divide_414c5/1
  Constant_T_w_12eeb/1 -> Divide_414c5/2
  Divide_414c5/1 -> Add_91898/2
  Add_91898/1 -> Blockout_d_Px_1_SG_D_3_0a11a/1

== system IEEE9Buses/SG_D_3/d_Px_2_SG_D_3_block ==
  note: d_Px_2_SG_D_3 in SG9
      | $\frac{\mathrm{Px}_{1,\mathrm{SG},D,3}-T_{2}\,\left(\frac{\mathrm{Px}_{1,\mathrm{SG},D,3}}{T_{w}}-\frac{w_{\mathrm{SG},D,3}-2\,\pi \,f_{0}}{T_{w}}\right)}{T_{1}}-\frac{\mathrm{Px}_{2,\mathrm{SG},D,3}}{T_{1}}$
      | Automatically generated on 2025-09-12 21:33:47 .
  State_Px_2_SG_D_3_70e41 : Inport
  State_Px_1_SG_D_3_ddb4e : Inport  Port=2
  State_Px_1_SG_D_3_337bf : Inport  Port=3
  State_w_SG_D_3_8dc04 : Inport  Port=4
  Add_40879 : Sum
  Add_4acb8 : Sum
  Add_60f53 : Sum
  Add_f1a91 : Sum
  Constant_-1_9df46 : Constant  Value=-1
  Constant_-1_a1892 : Constant  Value=-1
  Constant_-2.0_74665 : Constant  Value=-2.0
  Constant_T_1_d98c9 : Constant  Value=T_1
  Constant_T_1_ec95e : Constant  Value=T_1
  Constant_T_2_f537b : Constant  Value=T_2
  Constant_T_w_20ccb : Constant  Value=T_w
  Constant_T_w_59f88 : Constant  Value=T_w
  Constant_f0_d0c33 : Constant  Value=f0
  Constant_pi_a14ef : Constant  Value=pi
  Divide_00179 : Product  Inputs=*/
  Divide_05916 : Product  Inputs=*/
  Divide_1a984 : Product  Inputs=*/
  Divide_2a45f : Product  Inputs=*/
  Product_0e835 : Product
  Product_2fef7 : Product
  Product_50567 : Product
  Product_7538a : Product
  Product_ddd0c : Product
  Blockout_d_Px_2_SG_D_3_19155 : Outport
  wires:
  State_Px_1_SG_D_3_337bf/1 -> Product_50567/2
  Constant_-2.0_74665/1 -> Product_0e835/1
  Constant_f0_d0c33/1 -> Product_7538a/2
  Constant_pi_a14ef/1 -> Product_0e835/2
  Product_0e835/1 -> Product_7538a/1
  State_w_SG_D_3_8dc04/1 -> Add_4acb8/2
  Constant_-1_9df46/1 -> Product_50567/1
  Product_7538a/1 -> Add_4acb8/1
  Product_50567/1 -> Divide_00179/1
  Constant_T_w_59f88/1 -> Divide_00179/2
  Add_4acb8/1 -> Divide_05916/1
  Constant_T_w_20ccb/1 -> Divide_05916/2
  Divide_00179/1 -> Add_40879/1
  Divide_05916/1 -> Add_40879/2
  Constant_T_2_f537b/1 -> Product_2fef7/1
  Add_40879/1 -> Product_2fef7/2
  Constant_-1_a1892/1 -> Product_ddd0c/1
  Product_2fef7/1 -> Add_60f53/2
  State_Px_2_SG_D_3_70e41/1 -> Product_ddd0c/2
  State_Px_1_SG_D_3_ddb4e/1 -> Add_60f53/1
  Product_ddd0c/1 -> Divide_2a45f/1
  Add_f1a91/1 -> Blockout_d_Px_2_SG_D_3_19155/1
  Constant_T_1_d98c9/1 -> Divide_2a45f/2
  Add_60f53/1 -> Divide_1a984/1
  Constant_T_1_ec95e/1 -> Divide_1a984/2
  Divide_2a45f/1 -> Add_f1a91/1
  Divide_1a984/1 -> Add_f1a91/2

== system IEEE9Buses/SG_D_3/d_Px_3_SG_D_3_block ==
  note: d_Px_3_SG_D_3 in SG9
      | $\frac{\mathrm{Px}_{2,\mathrm{SG},D,3}+T_{4}\,\left(\frac{\mathrm{Px}_{1,\mathrm{SG},D,3}-T_{2}\,\left(\frac{\mathrm{Px}_{1,\mathrm{SG},D,3}}{T_{w}}-\frac{w_{\mathrm{SG},D,3}-2\,\pi \,f_{0}}{T_{w}}\right)}{T_{1}}-\frac{\mathrm{Px}_{2,\mathrm{SG},D,3}}{T_{1}}\right)}{T_{3}}-\frac{\mathrm{Px}_{3,\mathrm{SG},D,3}}{T_{3}}$
      | Automatically generated on 2025-09-12 21:33:50 .
  State_Px_3_SG_D_3_d10c2 : Inport
  State_Px_2_SG_D_3_2a129 : Inport  Port=2
  State_Px_2_SG_D_3_4e92f : Inport  Port=3
  State_Px_1_SG_D_3_747be : Inport  Port=4
  State_Px_1_SG_D_3_3120b : Inport  Port=5
  State_w_SG_D_3_3061a : Inport  Port=6
  Add_55d28 : Sum
  Add_5b089 : Sum
  Add_77bb1 : Sum
  Add_8a934 : Sum
  Add_c2a0c : Sum
  Add_e5def : Sum
  Constant_-1_34caa : Constant  Value=-1
  Constant_-1_c7aa7 : Constant  Value=-1
  Constant_-1_c9a76 : Constant  Value=-1
  Constant_-2.0_9bd05 : Constant  Value=-2.0
  Constant_T_1_7d76f : Constant  Value=T_1
  Constant_T_1_bf990 : Constant  Value=T_1
  Constant_T_2_06de4 : Constant  Value=T_2
  Constant_T_3_afdeb : Constant  Value=T_3
  Constant_T_3_f2b9a : Constant  Value=T_3
  Constant_T_4_ac7bf : Constant  Value=T_4
  Constant_T_w_135af : Constant  Value=T_w
  Constant_T_w_b08be : Constant  Value=T_w
  Constant_f0_70136 : Constant  Value=f0
  Constant_pi_ef6a3 : Constant  Value=pi
  Divide_10d6b : Product  Inputs=*/
  Divide_3681a : Product  Inputs=*/
  Divide_6cba0 : Product  Inputs=*/
  Divide_ad4c0 : Product  Inputs=*/
  Divide_b0187 : Product  Inputs=*/
  Divide_b24d9 : Product  Inputs=*/
  Product_38e37 : Product
  Product_472c9 : Product
  Product_47427 : Product
  Product_4a2c1 : Product
  Product_63e5d : Product
  Product_781c2 : Product
  Product_826b2 : Product
  Blockout_d_Px_3_SG_D_3_77867 : Outport
  wires:
  State_Px_1_SG_D_3_3120b/1 -> Product_472c9/2
  Constant_f0_70136/1 -> Product_38e37/2
  Constant_-2.0_9bd05/1 -> Product_781c2/1
  Add_5b089/1 -> Divide_10d6b/1
  Constant_pi_ef6a3/1 -> Product_781c2/2
  Product_781c2/1 -> Product_38e37/1
  State_w_SG_D_3_3061a/1 -> Add_e5def/2
  Constant_T_w_b08be/1 -> Divide_b24d9/2
  Constant_-1_c9a76/1 -> Product_472c9/1
  Product_38e37/1 -> Add_e5def/1
  Product_472c9/1 -> Divide_b24d9/1
  Add_e5def/1 -> Divide_6cba0/1
  Product_4a2c1/1 -> Divide_ad4c0/1
  Constant_T_w_135af/1 -> Divide_6cba0/2
  Divide_b24d9/1 -> Add_c2a0c/1
  Divide_6cba0/1 -> Add_c2a0c/2
  Constant_T_2_06de4/1 -> Product_826b2/1
  Add_c2a0c/1 -> Product_826b2/2
  Constant_-1_c7aa7/1 -> Product_4a2c1/1
  State_Px_2_SG_D_3_4e92f/1 -> Product_4a2c1/2
  State_Px_1_SG_D_3_747be/1 -> Add_5b089/1
  Constant_T_3_f2b9a/1 -> Divide_3681a/2
  Product_826b2/1 -> Add_5b089/2
  Constant_T_1_7d76f/1 -> Divide_ad4c0/2
  Add_8a934/1 -> Product_47427/2
  Constant_T_1_bf990/1 -> Divide_10d6b/2
  Divide_b0187/1 -> Add_77bb1/2
  Divide_ad4c0/1 -> Add_8a934/1
  Divide_10d6b/1 -> Add_8a934/2
  Constant_T_4_ac7bf/1 -> Product_47427/1
  Constant_-1_34caa/1 -> Product_63e5d/1
  State_Px_3_SG_D_3_d10c2/1 -> Product_63e5d/2
  State_Px_2_SG_D_3_2a129/1 -> Add_55d28/1
  Product_47427/1 -> Add_55d28/2
  Product_63e5d/1 -> Divide_3681a/1
  Add_55d28/1 -> Divide_b0187/1
  Constant_T_3_afdeb/1 -> Divide_b0187/2
  Divide_3681a/1 -> Add_77bb1/1
  Add_77bb1/1 -> Blockout_d_Px_3_SG_D_3_77867/1

== system IEEE9Buses/SG_D_3/d_R_f_SG_D_3_block ==
  note: d_R_f_SG_D_3 in SG9
      | $-\frac{R_{f,\mathrm{SG},D,3}-\frac{E_{\mathrm{fd},\mathrm{SG},D,3}\,K_{F}}{T_{F}}}{T_{F}}$
      | Automatically generated on 2025-09-12 21:33:43 .
  State_E_fd_SG_D_3_87a80 : Inport
  State_R_f_SG_D_3_37387 : Inport  Port=2
  Constant_K_F_838d0 : Constant  Value=K_F
  Constant_T_F_61e1e : Constant  Value=T_F
  Constant_T_F_a5385 : Constant  Value=T_F
  Divide_24b06 : Product  Inputs=*/
  Divide_fbb9b : Product  Inputs=*/
  Product_1d673 : Product
  Subtract_beafc : Sum  Inputs=+-
  Blockout_d_R_f_SG_D_3_9bb7b : Outport
  wires:
  State_E_fd_SG_D_3_87a80/1 -> Product_1d673/1
  Constant_T_F_a5385/1 -> Divide_24b06/2
  Constant_K_F_838d0/1 -> Product_1d673/2
  Product_1d673/1 -> Divide_24b06/1
  Divide_24b06/1 -> Subtract_beafc/1
  State_R_f_SG_D_3_37387/1 -> Subtract_beafc/2
  Subtract_beafc/1 -> Divide_fbb9b/1
  Constant_T_F_61e1e/1 -> Divide_fbb9b/2
  Divide_fbb9b/1 -> Blockout_d_R_f_SG_D_3_9bb7b/1

== system IEEE9Buses/SG_D_3/d_T_m_SG_D_3_block ==
  note: d_T_m_SG_D_3 in SG9
      | $-\frac{T_{m,\mathrm{SG},D,3}-T_{0}+\frac{\mathrm{SpeedPara}\,\left(w_{\mathrm{SG},D,3}-w_{\mathrm{ref}}\right)}{2\,f_{0}\,\pi }}{T_{\mathrm{speed}}}$
      | Automatically generated on 2025-09-12 21:33:34 .
  State_w_SG_D_3_82c70 : Inport
  State_T_m_SG_D_3_51fff : Inport  Port=2
  Add_2e6db : Sum
  Add_dfcb7 : Sum
  Constant_-1_ddc15 : Constant  Value=-1
  Constant_2.0_c8e07 : Constant  Value=2.0
  Constant_SpeedPara_b8988 : Constant  Value=SpeedPara
  Constant_T_0_c3849 : Constant  Value=T_0
  Constant_T_speed_08840 : Constant  Value=T_speed
  Constant_f0_9f69e : Constant  Value=f0
  Constant_pi_f3ca8 : Constant  Value=pi
  Constant_w_ref_6f00b : Constant  Value=w_ref
  Divide_01770 : Product  Inputs=*/
  Divide_0f3c5 : Product  Inputs=*/
  Product_02631 : Product
  Product_28ce6 : Product
  Product_90610 : Product
  Product_fb62c : Product
  Subtract_965ca : Sum  Inputs=+-
  Blockout_d_T_m_SG_D_3_5c1e7 : Outport
  wires:
  Constant_SpeedPara_b8988/1 -> Product_02631/1
  Constant_-1_ddc15/1 -> Product_90610/1
  Constant_w_ref_6f00b/1 -> Add_2e6db/2
  State_w_SG_D_3_82c70/1 -> Product_90610/2
  Constant_2.0_c8e07/1 -> Product_fb62c/1
  Product_90610/1 -> Add_2e6db/1
  Constant_pi_f3ca8/1 -> Product_fb62c/2
  Add_2e6db/1 -> Product_02631/2
  Product_fb62c/1 -> Product_28ce6/1
  Constant_f0_9f69e/1 -> Product_28ce6/2
  Product_02631/1 -> Divide_0f3c5/1
  Product_28ce6/1 -> Divide_0f3c5/2
  Divide_0f3c5/1 -> Add_dfcb7/1
  Constant_T_0_c3849/1 -> Add_dfcb7/2
  Add_dfcb7/1 -> Subtract_965ca/1
  State_T_m_SG_D_3_51fff/1 -> Subtract_965ca/2
  Subtract_965ca/1 -> Divide_01770/1
  Constant_T_speed_08840/1 -> Divide_01770/2
  Divide_01770/1 -> Blockout_d_T_m_SG_D_3_5c1e7/1
